simulink model "course_loop"  (Simulink 8.0)
settings: Solver=ode45  StartTime=0.0  StopTime=100  RelTol=1e-3
values from neighbouring files (symbols this model uses):
  phi_max = 15*pi/180    (= 0.261799387799)    [computeGains.m]
undefined symbols (not defined in the file or in its folder): P
settings Model: Creator=beard  LastModifiedBy=Gary
settings DataIOCC: SignalLoggingSaveFormat=ModelDataLogs
settings DebuggingCC: FcnCallInpInsideContextMsg=UseLocalSettings  StrictBusMsg=Warning
settings GRTTargetCC: CombineOutputUpdateFcns=off  GRTInterface=on

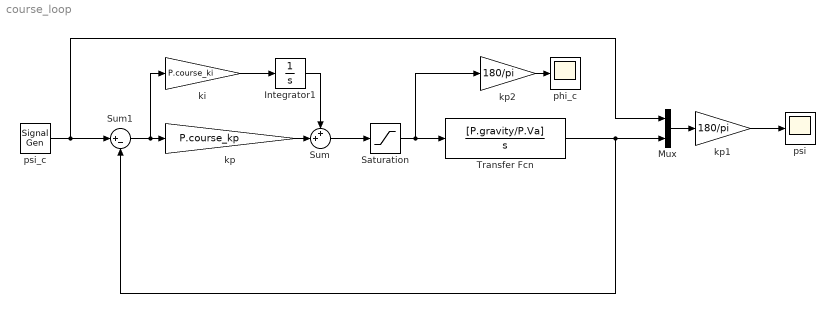
== system course_loop ==
  Integrator1 : Integrator
  Mux : Mux  Inputs=2
  Saturation : Saturate  UpperLimit=phi_max  LowerLimit=-phi_max
  Sum : Sum  Inputs=++|
  Sum1 : Sum  Inputs=|+-
  Transfer Fcn : TransferFcn  Numerator=[P.gravity/P.Va]  Denominator=[1 0]
  ki : Gain  Gain=P.course_ki
  kp : Gain  Gain=P.course_kp
  kp1 : Gain  Gain=180/pi
  kp2 : Gain  Gain=180/pi
  phi_c : Scope
      settings: TimeRange=100  YMin=-30  YMax=30
  psi : Scope
      settings: TimeRange=100  YMin=-100  YMax=100
  psi_c : SignalGenerator  WaveForm=square  Amplitude=25*pi/180  Frequency=.02
  wires:
  Transfer Fcn/1 -> Sum1/2, Mux/2
  Saturation/1 -> Transfer Fcn/1, kp2/1
  Sum/1 -> Saturation/1
  kp/1 -> Sum/2
  Sum1/1 -> kp/1, ki/1
  ki/1 -> Integrator1/1
  Integrator1/1 -> Sum/1
  psi_c/1 -> Sum1/1, Mux/1
  kp1/1 -> psi/1
  Mux/1 -> kp1/1
  kp2/1 -> phi_c/1
